simulink model "problem_2"  (R2020b)
settings: Solver=VariableStepAuto  StartTime=0.0  StopTime=100  RelTol=1e-3
model workspace (MAT data in the model file):
  b = Simulink.Parameter
  b.Value = 290
  b.DataType = 'auto'
  b.Dimensions = [1 1]
  k1 = Simulink.Parameter
  k1.Value = 5700
  k1.DataType = 'auto'
  k1.Dimensions = [1 1]
  k2 = Simulink.Parameter
  k2.Value = 135
  k2.DataType = 'auto'
  k2.Dimensions = [1 1]
  m1 = Simulink.Parameter
  m1.Value = 465
  m1.DataType = 'auto'
  m1.Dimensions = [1 1]
  m2 = Simulink.Parameter
  m2.Value = 50
  m2.DataType = 'auto'
  m2.Dimensions = [1 1]
settings Model: Creator=k.Raviteja  LastModifiedBy=k.Raviteja

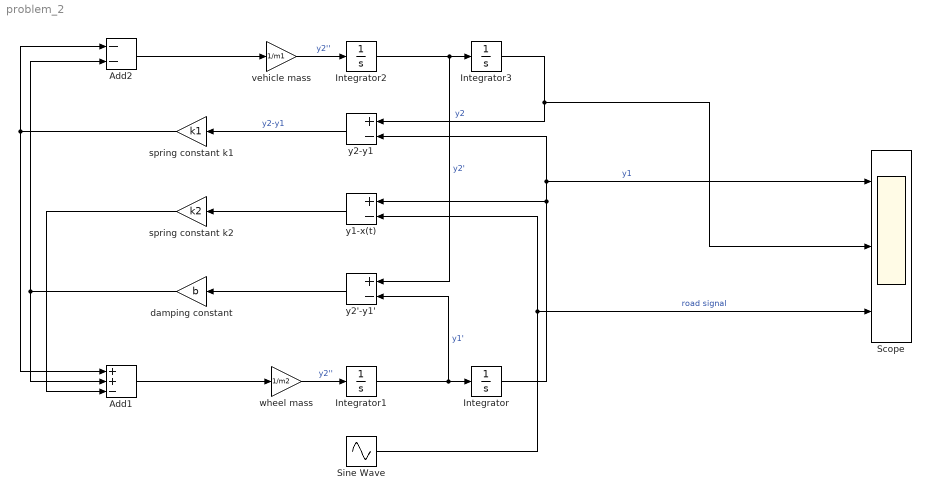
== system problem_2 ==
  Add1 : Sum  Inputs=++-
  Add2 : Sum  Inputs=--
  Integrator{,1..3} (4 alike) : Integrator
  Scope : Scope  NumInputPorts=3
  Sine Wave : Sin  SampleTime=0
  damping constant : Gain  Gain=b
  spring constant k1 : Gain  Gain=k1
  spring constant k2 : Gain  Gain=k2
  vehicle mass : Gain  Gain=1/m1
  wheel mass : Gain  Gain=1/m2
  y1-x(t) : Sum  Inputs=+-
  y2'-y1' : Sum  Inputs=+-
  y2-y1 : Sum  Inputs=+-
  wires:
  Integrator2/1 -> y2'-y1'/1, Integrator3/1  "y2'"
  Integrator1/1 -> y2'-y1'/2, Integrator/1  "y1'"
  Integrator3/1 -> Scope/2, y2-y1/1  "y2"
  Integrator/1 -> Scope/1, y2-y1/2, y1-x(t)/1  "y1"
  vehicle mass/1 -> Integrator2/1  "y2''"
  wheel mass/1 -> Integrator1/1  "y2''"
  Add2/1 -> vehicle mass/1
  Add1/1 -> wheel mass/1
  y2-y1/1 -> spring constant k1/1  "y2-y1"
  y2'-y1'/1 -> damping constant/1
  Sine Wave/1 -> Scope/3, y1-x(t)/2  "road signal"
  y1-x(t)/1 -> spring constant k2/1
  spring constant k1/1 -> Add1/1, Add2/1
  damping constant/1 -> Add1/2, Add2/2
  spring constant k2/1 -> Add1/3
